simulink model "poc_new_ut"  (Simulink 8.1)
settings: Solver=FixedStepDiscrete  StartTime=0.0  StopTime=10.0  FixedStep=5e-3  RelTol=1e-3
libraries: siltestlib x6, idiada_lib x5, poc_new x1
settings Model: Creator=xsellart  LastModifiedBy=AT015555
settings DataIOCC: SignalLoggingSaveFormat=Dataset
settings OptimizationCC: ExpressionDepthLimit=128
settings DebuggingCC: FcnCallInpInsideContextMsg=EnableAllAsError
settings GRTTargetCC: CombineOutputUpdateFcns=on  GRTInterface=off

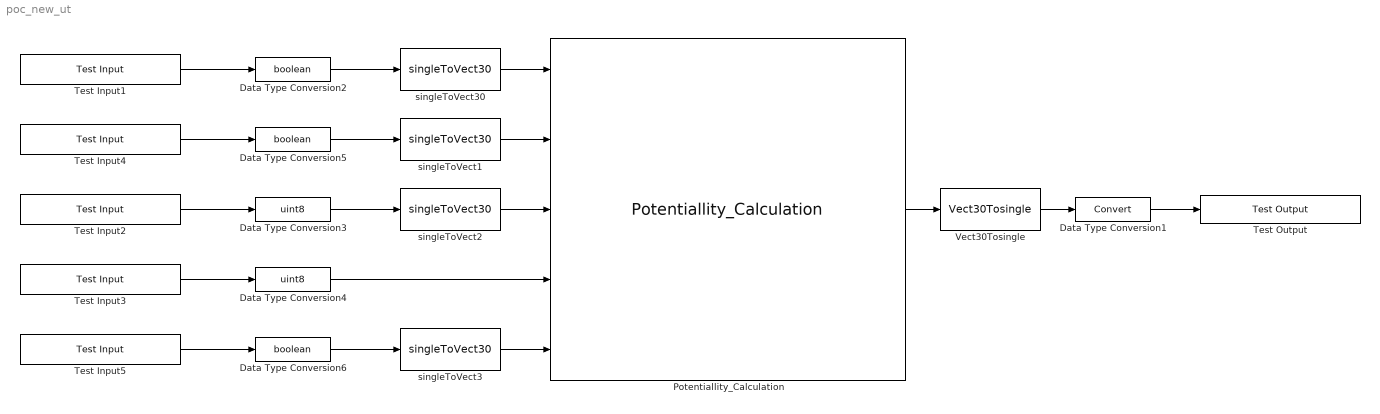
== system poc_new_ut ==
  Data Type Conversion1 : DataTypeConversion
  Data Type Conversion2 : DataTypeConversion  OutDataTypeStr=boolean
  Data Type Conversion3 : DataTypeConversion  OutDataTypeStr=uint8
  Data Type Conversion4 : DataTypeConversion  OutDataTypeStr=uint8
  Data Type Conversion5 : DataTypeConversion  OutDataTypeStr=boolean
  Data Type Conversion6 : DataTypeConversion  OutDataTypeStr=boolean
  Potentiallity_Calculation : poc_new/Potentiallity_Calculation
  Test Input1 : siltestlib/Test Input  varname=VIFO_PosCentralCrashVect30_flg  sampletime=-1
  Test Input2 : siltestlib/Test Input  varname=VPER_TargIdVect30_num  sampletime=-1
  Test Input3 : siltestlib/Test Input  varname=VPER_NumberOfTargets_enum  sampletime=-1
  Test Input4 : siltestlib/Test Input  varname=VIFO_PosLateralCrashVect30_flg  sampletime=-1
  Test Input5 : siltestlib/Test Input  varname=VIFO_AEBVehInPathVect30_flg  sampletime=-1
  Test Output : siltestlib/Test Output  varname=VIFO_PotentiallityVect30_perc  sampletime=-1
  Vect30Tosingle : idiada_lib/Vect30Tosingle
  singleToVect{1..3,30} (4 alike) : idiada_lib/singleToVect30
  wires:
  Potentiallity_Calculation/1 -> Vect30Tosingle/1
  Data Type Conversion1/1 -> Test Output/1
  Test Input1/1 -> Data Type Conversion2/1
  Data Type Conversion2/1 -> singleToVect30/1
  Test Input2/1 -> Data Type Conversion3/1
  Data Type Conversion3/1 -> singleToVect2/1
  Test Input3/1 -> Data Type Conversion4/1
  Data Type Conversion4/1 -> Potentiallity_Calculation/4
  Test Input4/1 -> Data Type Conversion5/1
  Data Type Conversion5/1 -> singleToVect1/1
  Test Input5/1 -> Data Type Conversion6/1
  Data Type Conversion6/1 -> singleToVect3/1
  singleToVect30/1 -> Potentiallity_Calculation/1
  singleToVect1/1 -> Potentiallity_Calculation/2
  singleToVect2/1 -> Potentiallity_Calculation/3
  singleToVect3/1 -> Potentiallity_Calculation/5
  Vect30Tosingle/1 -> Data Type Conversion1/1
